simulink model "inlamningregler21"  (R2016b)
settings: Solver=VariableStepAuto  StartTime=0.0  StopTime=2000  RelTol=1e-3
settings Model: Creator=mikpau  LastModifiedBy=mikpau

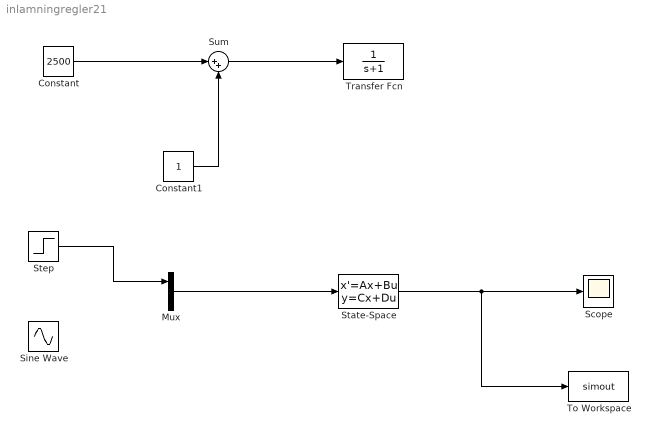
== system inlamningregler21 ==
  Constant : Constant  Value=2500
  Constant1 : Constant
  Mux : Mux  Inputs=2
  Scope : Scope
  Sine Wave : Sin  SampleTime=0
  State-Space : StateSpace  A=-0.0035  B=[1/2000, 0.0035]  D=[0, 0]  X0=0
  Step : Step  After=2500  SampleTime=0
  Sum : Sum  Inputs=|++
  To Workspace : ToWorkspace  VariableName=simout  SaveFormat=Timeseries  SampleTime=-1
  Transfer Fcn : TransferFcn  Denominator=[1 1]
  wires:
  Sum/1 -> Transfer Fcn/1
  Constant/1 -> Sum/1
  Constant1/1 -> Sum/2
  Step/1 -> Mux/1
  Mux/1 -> State-Space/1
  State-Space/1 -> To Workspace/1, Scope/1
